simulink model "receiver_202"  (R2022a)
settings: Solver=FixedStepAuto  StartTime=0.0  StopTime=10.0  RelTol=1e-3
libraries: androiduilib x3, androidaudiovideolib x1, androidcommunicationlib x1
settings Model: Creator=mohit  LastModifiedBy=Pratyaksh Bhayre
settings OptimizationCC: EnhancedBackFolding=on  PassReuseOutputArgsThreshold=0  MaxStackSize=64  OptimizeBlockOrder=speed  DifferentSizesBufferReuse=on  OptimizationCustomize=off
settings DebuggingCC: ParameterTunabilityLossMsg=error
settings HardwareCC: ProdBitPerLong=64  ProdLargestAtomicInteger=LongLong  ProdLargestAtomicFloat=Double  ProdLongLongMode=on  ProdHWDeviceType=ARM Compatible->ARM Cortex-A (64-bit)  UseEmbeddedCoderFeatures=off  UseSimulinkCoderFeatures=off
settings ModelReferenceCC: EnableRefExpFcnMdlSchedulingChecks=off
settings SFSimCC: MATLABDynamicMemAlloc=off
settings RTWCC: SystemTargetFile=ert.tlc  HardwareBoard=Android Device (64bit)  TLCOptions="-aInlineSetEventsForThisBaseRateFcn=TLC_FALSE -aSuppressMultiTaskScheduler=TLC_FALSE  -aRateBasedStepFcn=0"  TemplateMakefile=ert_default_tmf  RTWVerbose=off  Toolchain=Android SDK/NDK Tools
settings CodeAppCC: ForceParamTrailComments=on  OperatorAnnotations=on
settings ERTTargetCC: ERTCustomFileBanners=off  SupportContinuousTime=on  SupportNonInlinedSFcns=on  RemoveResetFunc=off  ModelStepFunctionPrototypeControlCompliant=off

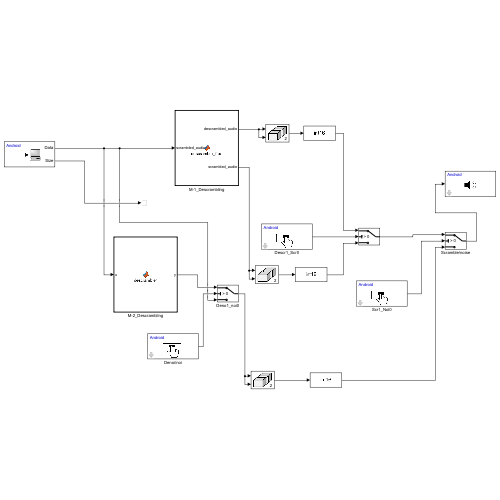
[thumbnail: Simulink's stored preview of the top-level diagram]
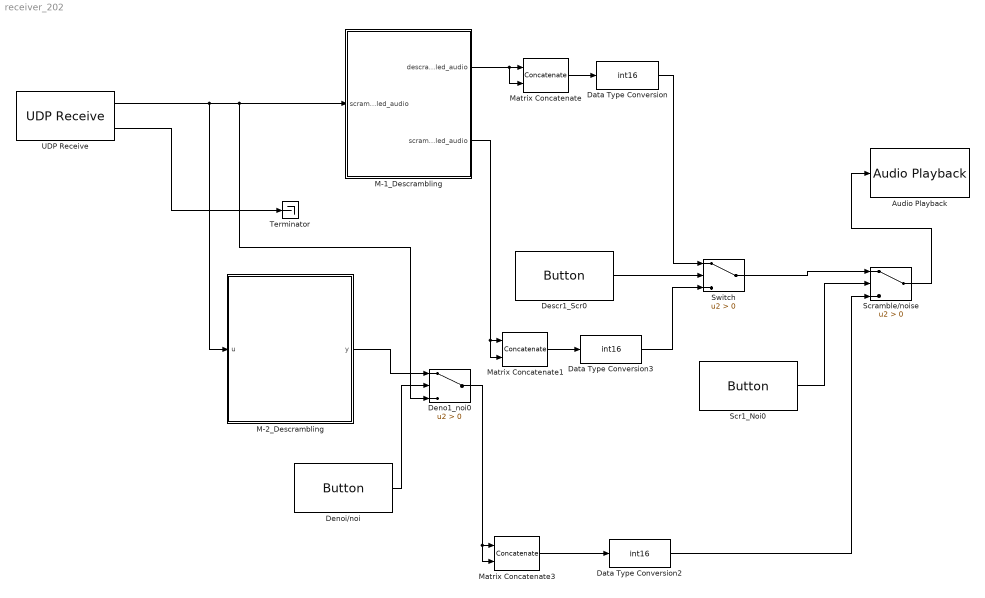
== system receiver_202 ==
  Audio Playback : androidaudiovideolib/Audio Playback  SampleFreq=44100  AudioSamplingFreq=44100  SampleTime=0.1  DeviceStr=0  QueueDuration=0  BlockPlatform=Android
      settings: SourceProductBaseCode=ANDROID
  Data Type Conversion : DataTypeConversion  OutDataTypeStr=int16  SaturateOnIntegerOverflow=off  RndMeth=Floor
  Data Type Conversion2 : DataTypeConversion  OutDataTypeStr=int16  SaturateOnIntegerOverflow=off  RndMeth=Floor
  Data Type Conversion3 : DataTypeConversion  OutDataTypeStr=int16  SaturateOnIntegerOverflow=off  RndMeth=Floor
  Deno1_noi0 : Switch  Criteria=u2 > Threshold  SaturateOnIntegerOverflow=off  InputSameDT=off
  Denoi/noi : androiduilib/Button  ButtonState=Not pressed  ButtonId=receiver_202/Denoi//noi  State=off  SampleTime=0.1  BlockPlatform=Android
      settings: SourceProductBaseCode=ANDROID
  Descr1_Scr0 : androiduilib/Button  ButtonState=Not pressed  ButtonId=receiver_202/Descr1_Scr0  State=off  SampleTime=0.1  BlockPlatform=Android
      settings: SourceProductBaseCode=ANDROID
  M-1_Descrambling : MATLAB Function  TreatAsAtomicUnit=on
  M-2_Descrambling : MATLAB Function  TreatAsAtomicUnit=on
  Matrix Concatenate : Concatenate  Mode=Multidimensional array  ConcatenateDimension=2
  Matrix Concatenate1 : Concatenate  Mode=Multidimensional array  ConcatenateDimension=2
  Matrix Concatenate3 : Concatenate  Mode=Multidimensional array  ConcatenateDimension=2
  Scr1_Noi0 : androiduilib/Button  ButtonState=Not pressed  ButtonId=receiver_202/Scr1_Noi0  State=off  SampleTime=0.1  BlockPlatform=Android
      settings: SourceProductBaseCode=ANDROID
  Scramble/noise : Switch  Criteria=u2 > Threshold  SaturateOnIntegerOverflow=off  InputSameDT=off
  Switch : Switch  Criteria=u2 > Threshold  SaturateOnIntegerOverflow=off  InputSameDT=off
  Terminator : Terminator
  UDP Receive : androidcommunicationlib/UDP Receive  localURL='0.0.0.0'  localPort=35000  remoteURL='0.0.0.0'  remotePort=-1  recvBufferSize=8192  signalDatatype=int16  dims=2205  isVarSize=off  showBlockingTime=off  blockingTime=0  sampletime=0.05  blockPlatform=Android
      settings: SourceProductBaseCode=ANDROID
  wires:
  UDP Receive/2 -> Terminator/1
  M-1_Descrambling/1(descrambled_audio) -> Matrix Concatenate/2, Matrix Concatenate/1
  Matrix Concatenate/1 -> Data Type Conversion/1
  Descr1_Scr0/1 -> Switch/2
  UDP Receive/1 -> Deno1_noi0/3, M-1_Descrambling/1("scrambled_audio "), M-2_Descrambling/1(u)
  M-1_Descrambling/2(scrambled_audio) -> Matrix Concatenate1/2, Matrix Concatenate1/1
  Data Type Conversion/1 -> Switch/1
  Matrix Concatenate3/1 -> Data Type Conversion2/1
  Matrix Concatenate1/1 -> Data Type Conversion3/1
  Data Type Conversion3/1 -> Switch/3
  Switch/1 -> Scramble/noise/1
  Scramble/noise/1 -> Audio Playback/1
  Scr1_Noi0/1 -> Scramble/noise/2
  M-2_Descrambling/1(y) -> Deno1_noi0/1
  Denoi/noi/1 -> Deno1_noi0/2
  Deno1_noi0/1 -> Matrix Concatenate3/2, Matrix Concatenate3/1
  Data Type Conversion2/1 -> Scramble/noise/3

== matlab function receiver_202/M-2_Descrambling ==
  data: u input; y output
function y = descrambler(u)
    % Extract the first channel of the input matrix (assuming u is Nx2)
    u = u(:,1);

    % Define the bucket size
    bucketSize = 20;

    % Perform FFT on the entire signal
    fftResult = fft(u);
    
    % Number of buckets in the entire signal
    numBuckets = floor(length(fftResult) / bucketSize);

    % Subtract the exact noise added during scrambling
    for i = 1:numBuckets
        % Define the range of indices for this bucket
        bucketStartIdx = (i-1) * bucketSize + 1;
        bucketEndIdx = bucketStartIdx + bucketSize - 1;

        % Remove noise from each element in the bucket
        for idx = bucketStartIdx:bucketEndIdx
            noise = (idx +10) * 1e6;  % Calculate noise as index * 10,00,000
            fftResult(idx) = fftResult(idx) - noise;  % Remove noise from positive frequency
            fftResult(end - idx + 2) = fftResult(end - idx + 2) - noise;  % Remove noise from negative frequency
        end
    end

    % Handle any remaining elements outside of full buckets
    if mod(length(fftResult), bucketSize) ~= 0
        remainingStart = numBuckets * bucketSize + 1;
        for idx = remainingStart:length(fftResult)
            noise = (idx+10) * 1e6;  % Calculate noise as index * 10,00,000
            fftResult(idx) = fftResult(idx) - noise;  % Remove noise from positive frequency
            fftResult(end - idx + 2) = fftResult(end - idx + 2) - noise;  % Remove noise from negative frequency
        end
    end

    % Enforce conjugate symmetry on fftResult to ensure real output from ifft
    N = length(fftResult);
    fftResult(2:N/2) = conj(fftResult(N:-1:N/2+2));

    % Perform the inverse FFT to get the descrambled time-domain signal
    descrambledChannel = ifft(fftResult);

    % Take the real part to ensure the output is real-valued
    y = real(descrambledChannel);
end

== matlab function receiver_202/M-1_Descrambling ==
  data: scrambled_audio input; descrambled_audio output; scrambled_audio output
function [descrambled_audio,scrambled_audio] = descramble_freq(scrambled_audio)
    % Descramble the scrambled audio input in the frequency domain using the same seed
    % scrambled_audio: [nx2] scrambled audio array
    % seed: The same integer seed used during scrambling
    seed=123;
    % Pre-allocate descrambled_audio array
    descrambled_audio = zeros(size(scrambled_audio));

    % Set the random seed to regenerate the same permutation
    rng(seed, 'twister');
    
    % Generate the same random permutation as scrambling
    n = size(scrambled_audio, 1);
%     swap_indices = perm(n);
    swap_indices = bitrevorder(1:n);
    scrambled_audio=scrambled_audio(:,1);
    % Apply FFT to each channel separately
    scrambled_freq_left = fft(scrambled_audio(:,1));
    %scrambled_freq_right = fft(scrambled_audio(:,2));

    % Reverse the swapping using the inverse of swap_indices
    inverse_indices = swap_indices;
    descrambled_freq_left = scrambled_freq_left(inverse_indices);
    %descrambled_freq_right = scrambled_freq_right(inverse_indices);

    % Convert back to time domain
    descrambled_audio(:,1) = real(ifft(descrambled_freq_left));
    %descrambled_audio(:,2) = real(ifft(descrambled_freq_right));
end
